simulink model "projeto"  (R2015a)
settings: Solver=FixedStepDiscrete  SolverMode=SingleTasking  StartTime=0.0  StopTime=inf  RelTol=1e-3
values from neighbouring files (symbols this model uses):
  delay_c1 = 24    [valores.m]
  delay_c2 = 24    [valores.m]
  delay_c3 = 28    [valores.m]
  delay_c4 = 31    [valores.m]
  delay_l1 = 12    [valores.m]
  delay_l4 = 5    [valores.m]
libraries: dsparch4 x19, commnoisgen2 x2, dspvision x2
settings Model: Creator=aluno  LastModifiedBy=moecke
settings DataIOCC: SaveOutput=off  SignalLogging=off  SaveTime=off
settings DebuggingCC: AlgebraicLoopMsg=error  SingleTaskRateTransMsg=error

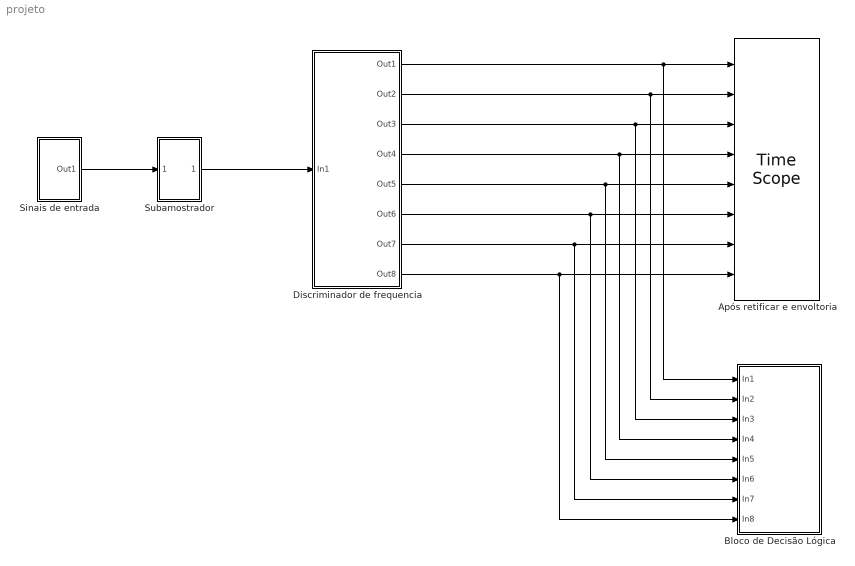
== system projeto ==
  Após retificar e envoltoria : TimeScope  DefaultConfigurationName=spbscopes.TimeScopeBlockCfg  NumInputPorts=8
  "Bloco de Decisão Lógica " : Subsystem
  Discriminador de frequencia : Subsystem
  Sinais de entrada : Subsystem
  Subamostrador : Subsystem
  wires:
  Discriminador de frequencia/1(Out1) -> "Bloco de Decisão Lógica "/1(In1), Após retificar e envoltoria/1
  Discriminador de frequencia/2(Out2) -> "Bloco de Decisão Lógica "/2(In2), Após retificar e envoltoria/2
  Discriminador de frequencia/3(Out3) -> "Bloco de Decisão Lógica "/3(In3), Após retificar e envoltoria/3
  Discriminador de frequencia/4(Out4) -> "Bloco de Decisão Lógica "/4(In4), Após retificar e envoltoria/4
  Discriminador de frequencia/5(Out5) -> "Bloco de Decisão Lógica "/5(In5), Após retificar e envoltoria/5
  Discriminador de frequencia/6(Out6) -> "Bloco de Decisão Lógica "/6(In6), Após retificar e envoltoria/6
  Discriminador de frequencia/7(Out7) -> "Bloco de Decisão Lógica "/7(In7), Após retificar e envoltoria/7
  Discriminador de frequencia/8(Out8) -> "Bloco de Decisão Lógica "/8(In8), Após retificar e envoltoria/8
  Subamostrador/1(Out1) -> Discriminador de frequencia/1(In1)
  Sinais de entrada/1(Out1) -> Subamostrador/1(In1)

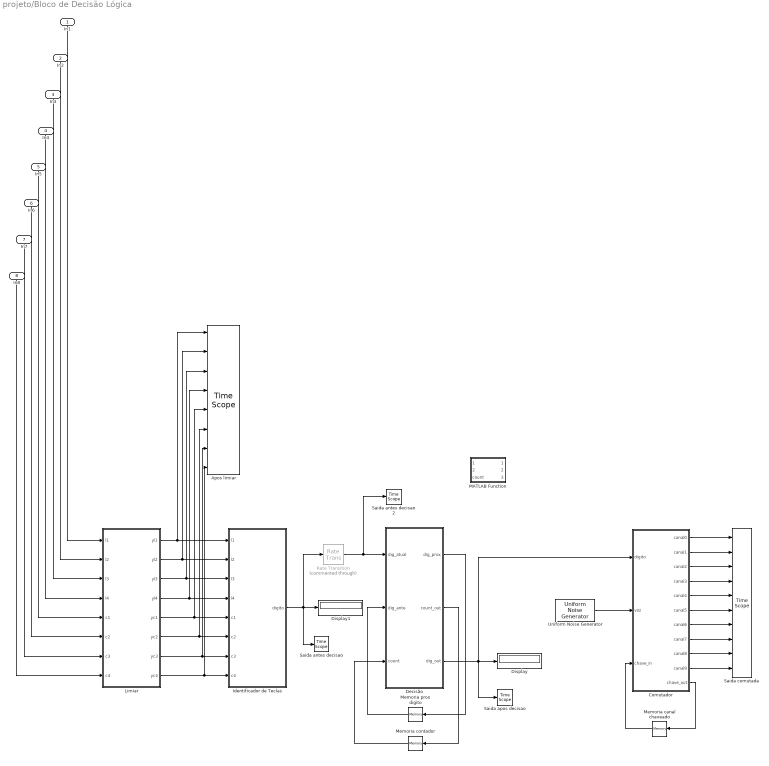
== system projeto/Bloco de Decisão Lógica  ==
  In1 : Inport
  In2 : Inport  Port=2
  In3 : Inport  Port=3
  In4 : Inport  Port=4
  In5 : Inport  Port=5
  In6 : Inport  Port=6
  In7 : Inport  Port=7
  In8 : Inport  Port=8
  Apos limiar : TimeScope  DefaultConfigurationName=spbscopes.TimeScopeBlockCfg  NumInputPorts=8
  Comutador : MATLAB Function  TreatAsAtomicUnit=on
  Decisão : MATLAB Function  TreatAsAtomicUnit=on
  Display : Display
  Display1 : Display
  Identificador de Teclas : MATLAB Function  TreatAsAtomicUnit=on
  Limiar : MATLAB Function  TreatAsAtomicUnit=on
  MATLAB Function : MATLAB Function  TreatAsAtomicUnit=on
  Memoria canal chaveado : Memory
  Memoria contador : Memory
  Memoria prox digito : Memory
  Rate Transition : RateTransition  Commented=through  Deterministic=off  OutPortSampleTime=0
  Saida antes decisao : TimeScope  DefaultConfigurationName=spbscopes.TimeScopeBlockCfg
  Saida antes decisao 2 : TimeScope  DefaultConfigurationName=spbscopes.TimeScopeBlockCfg
  Saida apos decisao : TimeScope  DefaultConfigurationName=spbscopes.TimeScopeBlockCfg
  Saida comutada : TimeScope  DefaultConfigurationName=spbscopes.TimeScopeBlockCfg  NumInputPorts=10
  Uniform Noise Generator : commnoisgen2/Uniform Noise Generator  low=-1  up=1  seed=31  Ts=1/44100  frameBased=off  sampPerFrame=1  orient=off  outDataType=double
  wires:
  In5/1 -> Limiar/5(c1)
  In6/1 -> Limiar/6(c2)
  In2/1 -> Limiar/2(l2)
  In1/1 -> Limiar/1(l1)
  Identificador de Teclas/1(digito) -> Display1/1, Saida antes decisao/1, Rate Transition/1
  In7/1 -> Limiar/7(c3)
  In3/1 -> Limiar/3(l3)
  In8/1 -> Limiar/8(c4)
  In4/1 -> Limiar/4(l4)
  Limiar/1(yl1) -> Identificador de Teclas/1(l1), Apos limiar/1
  Limiar/2(yl2) -> Identificador de Teclas/2(l2), Apos limiar/2
  Limiar/3(yl3) -> Identificador de Teclas/3(l3), Apos limiar/3
  Limiar/4(yl4) -> Identificador de Teclas/4(l4), Apos limiar/4
  Limiar/5(yc1) -> Identificador de Teclas/5(c1), Apos limiar/5
  Limiar/6(yc2) -> Identificador de Teclas/6(c2), Apos limiar/6
  Limiar/7(yc3) -> Identificador de Teclas/7(c3), Apos limiar/7
  Limiar/8(yc4) -> Identificador de Teclas/8(c4), Apos limiar/8
  Decisão/1(dig_prox) -> Memoria prox digito/1
  Memoria prox digito/1 -> Decisão/2(dig_ante)
  Decisão/2(count_out) -> Memoria contador/1
  Memoria contador/1 -> Decisão/3(count)
  Decisão/3(dig_out) -> Comutador/1(digito), Saida apos decisao/1, Display/1
  Rate Transition/1 -> Saida antes decisao 2/1, Decisão/1(dig_atual)
  Comutador/1(canal0) -> Saida comutada/1
  Comutador/2(canal1) -> Saida comutada/2
  Comutador/3(canal2) -> Saida comutada/3
  Comutador/4(canal3) -> Saida comutada/4
  Comutador/5(canal4) -> Saida comutada/5
  Comutador/6(canal5) -> Saida comutada/6
  Comutador/7(canal6) -> Saida comutada/7
  Comutador/8(canal7) -> Saida comutada/8
  Comutador/9(canal8) -> Saida comutada/9
  Comutador/10(canal9) -> Saida comutada/10
  Uniform Noise Generator/1 -> Comutador/2(voz)
  Comutador/11(chave_out) -> Memoria canal chaveado/1
  Memoria canal chaveado/1 -> Comutador/3(chave_in)

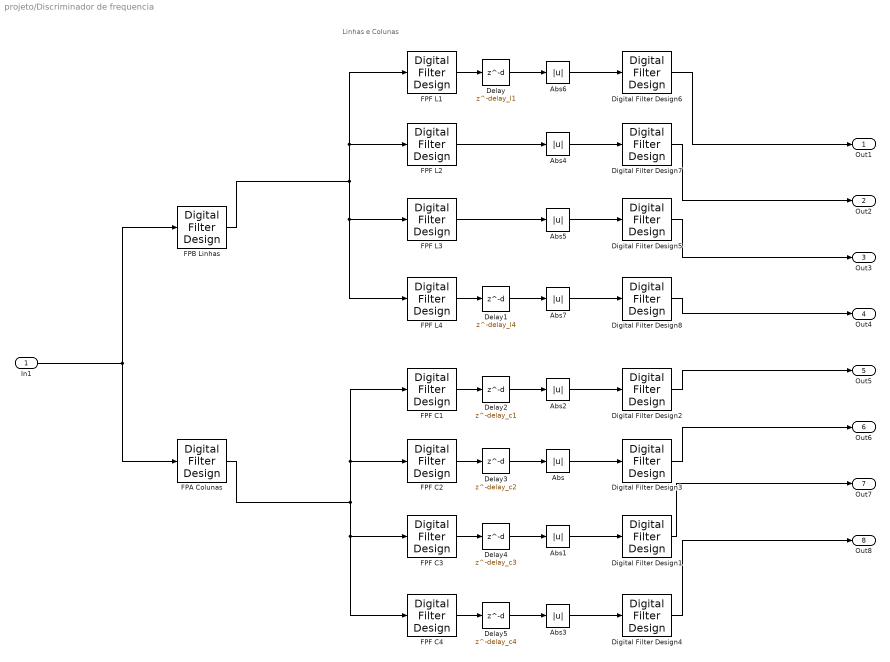
== system projeto/Discriminador de frequencia ==
  note: Linhas e Colunas
  In1 : Inport
  " FPF L3" : dsparch4/Digital Filter Design  mwdsp_browser_bugfix_var=off
  Abs{,1..7} (8 alike) : Abs
  Delay : Delay  DelayLength=delay_l1  InputProcessing=Columns as channels (frame based)
  Delay1 : Delay  DelayLength=delay_l4  InputProcessing=Columns as channels (frame based)
  Delay2 : Delay  DelayLength=delay_c1  InputProcessing=Columns as channels (frame based)
  Delay3 : Delay  DelayLength=delay_c2  InputProcessing=Columns as channels (frame based)
  Delay4 : Delay  DelayLength=delay_c3  InputProcessing=Columns as channels (frame based)
  Delay5 : Delay  DelayLength=delay_c4  InputProcessing=Columns as channels (frame based)
  Digital Filter Design{1..8} (8 alike) : dsparch4/Digital Filter Design  mwdsp_browser_bugfix_var=off
  FPA Colunas : dsparch4/Digital Filter Design  mwdsp_browser_bugfix_var=off
  FPB Linhas : dsparch4/Digital Filter Design  mwdsp_browser_bugfix_var=off
  FPF C{1..4} (4 alike) : dsparch4/Digital Filter Design  mwdsp_browser_bugfix_var=off
  FPF L1 : dsparch4/Digital Filter Design  mwdsp_browser_bugfix_var=off
  FPF L2 : dsparch4/Digital Filter Design  mwdsp_browser_bugfix_var=off
  FPF L4 : dsparch4/Digital Filter Design  mwdsp_browser_bugfix_var=off
  Out1 : Outport
  Out2 : Outport  Port=2
  Out3 : Outport  Port=3
  Out4 : Outport  Port=4
  Out5 : Outport  Port=5
  Out6 : Outport  Port=6
  Out7 : Outport  Port=7
  Out8 : Outport  Port=8
  wires:
  Digital Filter Design2/1 -> Out5/1
  Digital Filter Design7/1 -> Out2/1
  Digital Filter Design8/1 -> Out4/1
  Digital Filter Design5/1 -> Out3/1
  Digital Filter Design3/1 -> Out6/1
  Digital Filter Design1/1 -> Out7/1
  Digital Filter Design6/1 -> Out1/1
  In1/1 -> FPB Linhas/1, FPA Colunas/1
  FPA Colunas/1 -> FPF C1/1, FPF C2/1, FPF C4/1, FPF C3/1
  Digital Filter Design4/1 -> Out8/1
  FPF C2/1 -> Delay3/1
  FPF C3/1 -> Delay4/1
  FPF C1/1 -> Delay2/1
  Abs1/1 -> Digital Filter Design1/1
  Abs2/1 -> Digital Filter Design2/1
  Abs/1 -> Digital Filter Design3/1
  FPF C4/1 -> Delay5/1
  Abs3/1 -> Digital Filter Design4/1
  FPF L2/1 -> Abs4/1
  " FPF L3"/1 -> Abs5/1
  FPF L1/1 -> Delay/1
  Abs5/1 -> Digital Filter Design5/1
  Abs6/1 -> Digital Filter Design6/1
  Abs4/1 -> Digital Filter Design7/1
  FPF L4/1 -> Delay1/1
  Abs7/1 -> Digital Filter Design8/1
  FPB Linhas/1 -> FPF L4/1, " FPF L3"/1, FPF L2/1, FPF L1/1
  Delay/1 -> Abs6/1
  Delay1/1 -> Abs7/1
  Delay2/1 -> Abs2/1
  Delay3/1 -> Abs/1
  Delay4/1 -> Abs1/1
  Delay5/1 -> Abs3/1

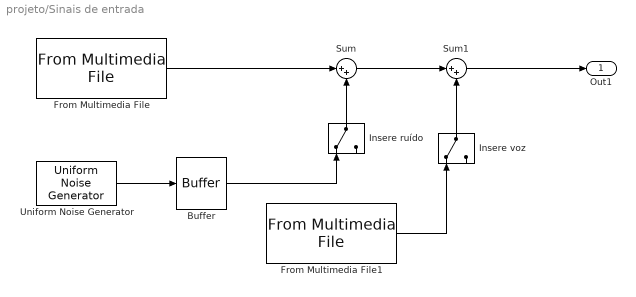
== system projeto/Sinais de entrada ==
  Buffer : Buffer  N=1024  TreatMby1Signals=One channel
  From Multimedia File : dspvision/From Multimedia File  inputFilename=DTMF65ms.wav  loop=on  numPlays=inf  outputStreams=Audio only  videoDataType=single  audioDataType=double  inheritSampleTime=on  userDefinedSampleTime=1/30  noAudioOutput=off  isIntensityVideo=off  fourcc=RGB  colorVideoFormat=Separate color signals  outputEOF=off  dataOrg=Column-major  audioFrameSize=1024  computeAudioFrameSize=off  outSamplingMode=Sample based
  From Multimedia File1 : dspvision/From Multimedia File  inputFilename=testando123.wav  loop=on  numPlays=inf  outputStreams=Audio only  videoDataType=single  audioDataType=double  inheritSampleTime=on  userDefinedSampleTime=1/30  noAudioOutput=off  isIntensityVideo=off  fourcc=RGB  colorVideoFormat=Separate color signals  outputEOF=off  dataOrg=Column-major  audioFrameSize=1024  computeAudioFrameSize=off  outSamplingMode=Sample based
  Insere ruído : ManualSwitch
  Insere voz : ManualSwitch
  Sum : Sum  Inputs=|++
  Sum1 : Sum  Inputs=|++
  Uniform Noise Generator : commnoisgen2/Uniform Noise Generator  low=-1  up=1  seed=31  Ts=1/44100  frameBased=off  sampPerFrame=1  orient=off  outDataType=double
  Out1 : Outport
  wires:
  Uniform Noise Generator/1 -> Buffer/1
  From Multimedia File/1 -> Sum/1
  Sum/1 -> Sum1/1
  Sum1/1 -> Out1/1
  Insere ruído/1 -> Sum/2
  Buffer/1 -> Insere ruído/1
  Insere voz/1 -> Sum1/2
  From Multimedia File1/1 -> Insere voz/1

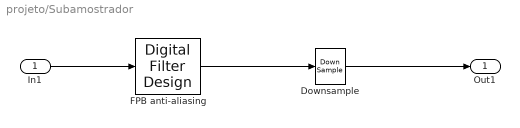
== system projeto/Subamostrador ==
  In1 : Inport
  " FPB anti-aliasing" : dsparch4/Digital Filter Design  mwdsp_browser_bugfix_var=off
  Downsample : DownSample  N=10  RateOptions=Allow multirate processing
  Out1 : Outport
  wires:
  Downsample/1 -> Out1/1
  In1/1 -> " FPB anti-aliasing"/1
  " FPB anti-aliasing"/1 -> Downsample/1

== matlab function projeto/Bloco de Decisão Lógica /Identificador de Teclas ==
  data: l1 input; digito output; l2 input; l3 input; l4 input; c1 input; c2 input; c3 input; c4 input
function digito = fcn(l1, l2, l3, l4, c1, c2, c3, c4)
%#codegen

for i = 1:length(l1)
    % Duas linhas ativadas ERRO2
    if (l1(i) && l2(i)) || (l1(i) && l3(i)) || (l1(i) && l3(i))
        digito = 14
    % Duas colunas ativadas ERRO3
    elseif (c1(i) && c2(i)) || (c1(i) && c3(i)) || (c1(i) && c3(i))
        digito = 15
    elseif l1(i) && c1(i)
        digito = 1;
    elseif l1(i) && c2(i)
        digito = 2;
    elseif l1(i) && c3(i)
        digito = 3;
    elseif l2(i) && c1(i)
        digito = 4;
    elseif l2(i) && c2(i)
        digito = 5;
    elseif l2(i) && c3(i)
        digito = 6;
    elseif l3(i) && c1(i)
        digito = 7;
    elseif l3(i) && c2(i)
        digito = 8;
    elseif l3(i) && c3(i)
        digito = 9;
    % Asterisco
    elseif l4(i) && c1(i)
        digito = 11;
    % Zero
    elseif l4(i) && c2(i)
        digito = 10;
    % Cerquilha
    elseif l4(i) && c3(i)
        digito = 12;
    % Codigo vazio
    else
        digito = 0;
    end
end

== matlab function projeto/Bloco de Decisão Lógica /Limiar ==
  data: l1 input; yl1 output; l2 input; l3 input; l4 input; c1 input; c2 input; c3 input; c4 input; yl2 output; yl3 output; yl4 output; yc1 output; yc2 output; yc3 output; yc4 output
function [yl1, yl2, yl3, yl4, yc1, yc2, yc3, yc4] = fcn(l1, l2, l3, l4, c1, c2, c3, c4)
%#codegen

limiar = 0.1;

linha1 = l1(1:end) > limiar;
linha2 = l2(1:end) > limiar;
linha3 = l3(1:end) > limiar;
linha4 = l4(1:end) > limiar;

coluna1 = c1(1:end) > limiar;
coluna2 = c2(1:end) > limiar;
coluna3 = c3(1:end) > limiar;
coluna4 = c4(1:end) > limiar;

% saidas
yl1 = linha1;
yl2 = linha2;
yl3 = linha3;
yl4 = linha4;
yc1 = coluna1;
yc2 = coluna2;
yc3 = coluna3;
yc4 = coluna4;

== matlab function projeto/Bloco de Decisão Lógica /Decisão ==
  data: dig_atual input; dig_prox output; dig_ante input; count input; count_out output; dig_out output
function [dig_prox, count_out, dig_out]= fcn(dig_atual, dig_ante, count)
%#codegen

n_20ms = 89; % Numero de amostras equivalente a 20 ms.

if (dig_atual == dig_ante)
    count_out = count + 1;
else
    count_out = 0;
end

if (count >= n_20ms)
    dig_out = dig_atual;
else
    dig_out = 0; % Vazio
end

 dig_prox = dig_atual;

== matlab function projeto/Bloco de Decisão Lógica /Comutador ==
  data: digito input; canal0 output; voz input; canal1 output; canal2 output; canal3 output; canal4 output; canal5 output; canal6 output; canal7 output; canal8 output; canal9 output; chave_in input; chave_out output
function [canal0, canal1, canal2, canal3, canal4, canal5, canal6, canal7, canal8, canal9, chave_out]= fcn(digito, voz, chave_in)
%#codegen
% canal0 = zeros(1024,1);
% canal1 = zeros(1024,1);
% canal2 = zeros(1024,1);
% canal3 = zeros(1024,1);
% canal4 = zeros(1024,1);
% canal5 = zeros(1024,1);
% canal6 = zeros(1024,1);
% canal7 = zeros(1024,1);
% canal8 = zeros(1024,1);
% canal9 = zeros(1024,1);

canal0 = 0;
canal1 = 0;
canal2 = 0;
canal3 = 0;
canal4 = 0;
canal5 = 0;
canal6 = 0;
canal7 = 0;
canal8 = 0;
canal9 = 0;

if chave_in == 0
    switch digito
       case 10
          canal0 = voz;
          chave_out = 10;
       case 1
          canal1 = voz;
          chave_out = 1;
       case 2
          canal2 = voz;
          chave_out = 2;
       case 3
          canal3 = voz;
          chave_out = 3;
       case 4
          canal4 = voz;
          chave_out = 4;
       case 5
          canal5 = voz;
          chave_out = 5;
       case 6
          canal6 = voz;
          chave_out = 6;
       case 7
          canal7 = voz;
          chave_out = 7;
       case 8
          canal8 = voz;
          chave_out = 8;
       case 9
          canal9 = voz;
          chave_out = 9;
        otherwise
          chave_out = 0;
    end
else
    switch chave_in
       case 10
          canal0 = voz;
       case 1
          canal1 = voz;
       case 2
          canal2 = voz;
       case 3
          canal3 = voz;
       case 4
          canal4 = voz;
       case 5
          canal5 = voz;
       case 6
          canal6 = voz;
       case 7
          canal7 = voz;
       case 8
          canal8 = voz;
       case 9
          canal9 = voz;
    end
    chave_out = chave_in;
end

== matlab function projeto/Bloco de Decisão Lógica /MATLAB Function ==
  data: dig_atual input; dig_prox output; dig_ante input; count input; count_out output; dig_out output
function [dig_prox, count_out, dig_out]= fcn(dig_atual, dig_ante, count)
%#codegen

n_20ms = 89; % Numero de amostras equivalente a 20 ms.

if (dig_atual == dig_ante)
    count_out = count + 1;
else
    count_out = 0;
end

if (count >= n_20ms)
    dig_out = dig_atual;
else
    dig_out = 0; % Vazio
end

 dig_prox = dig_atual;
